simulink model "my_dom_model_statyczne"  (R2018a)
settings: Solver=VariableStepAuto  StartTime=0.0  StopTime=10.0  RelTol=1e-3
values from neighbouring files (symbols this model uses):
  c_p = 1000    [leveled_NL.m]    (also in leveled_state_space.m; leveled_transmitancja.m; my_dom.m; my_dom_state_space_script.m)
  C_vp = c_p*ro_p*V_p    (= 120000)    [leveled_NL.m]    (also in leveled_state_space.m; leveled_transmitancja.m; my_dom.m; my_dom_state_space_script.m)
  C_vw = c_p*ro_p*V_w    (= 1200000)    [leveled_NL.m]    (also in leveled_state_space.m; leveled_transmitancja.m; my_dom.m; my_dom_state_space_script.m)
  K_1 = K_matrix(1,1)    [leveled_NL.m]    (also in leveled_state_space.m; leveled_transmitancja.m; my_dom.m; my_dom_state_space_script.m)
  K_p = p*K_w    [leveled_NL.m]    (also in leveled_state_space.m; leveled_transmitancja.m; my_dom.m; my_dom_state_space_script.m)
  K_w = K_matrix(2,1)    [leveled_NL.m]    (also in leveled_state_space.m; leveled_transmitancja.m; my_dom.m; my_dom_state_space_script.m)
  ro_p = 1.2    [leveled_NL.m]    (also in leveled_state_space.m; leveled_transmitancja.m; my_dom.m; my_dom_state_space_script.m)
  slope_f_p = 0    [my_dom_statyczne.m]
  slope_T_z = 0    [my_dom_statyczne.m]
  slope_T_zew = 0.00001    (= 1e-05)    [my_dom_statyczne.m]
  T_pN = 19    [leveled_NL.m]    (also in leveled_state_space.m; leveled_transmitancja.m; my_dom.m; my_dom_state_space_script.m)
  T_wewN = 21    [leveled_NL.m]    (also in leveled_state_space.m; leveled_transmitancja.m; my_dom.m; my_dom_state_space_script.m)
libraries: simulink x3
settings Model: Creator=johnb  LastModifiedBy=johnb

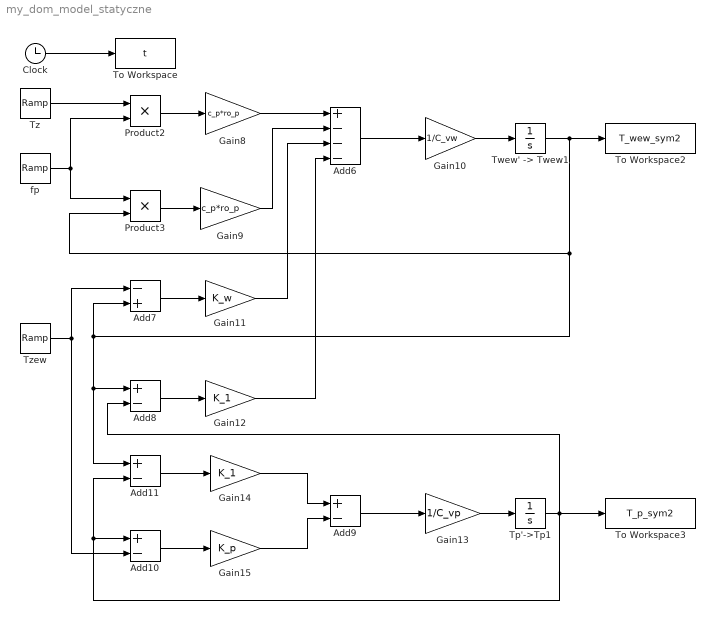
== system my_dom_model_statyczne ==
  Add{8..11} (4 alike) : Sum  Inputs=+-
  Add6 : Sum  Inputs=+---
  Add7 : Sum  Inputs=-+
  Clock : Clock
  Gain10 : Gain  Gain=1/C_vw
  Gain11 : Gain  Gain=K_w
  Gain12 : Gain  Gain=K_1
  Gain13 : Gain  Gain=1/C_vp
  Gain14 : Gain  Gain=K_1
  Gain15 : Gain  Gain=K_p
  Gain8 : Gain  Gain=c_p*ro_p
  Gain9 : Gain  Gain=c_p*ro_p
  Product2 : Product
  Product3 : Product
  To Workspace : ToWorkspace  VariableName=t  SampleTime=-1
  To Workspace2 : ToWorkspace  VariableName=T_wew_sym2  SampleTime=-1
  To Workspace3 : ToWorkspace  VariableName=T_p_sym2  SampleTime=-1
  Tp'->Tp1 : Integrator  InitialCondition=T_pN
  "Twew' -> Twew1" : Integrator  InitialCondition=T_wewN
  Tz : simulink/Sources/Ramp  slope=slope_T_z  start=0  InitialOutput=0
  Tzew : simulink/Sources/Ramp  slope=slope_T_zew  start=0  InitialOutput=0
  fp : simulink/Sources/Ramp  slope=slope_f_p  start=0  InitialOutput=0
  wires:
  Clock/1 -> To Workspace/1
  Gain12/1 -> Add6/4
  Add7/1 -> Gain11/1
  Gain13/1 -> Tp'->Tp1/1
  "Twew' -> Twew1"/1 -> To Workspace2/1, Add11/1, Add8/1, Add7/2, Product3/2
  Add8/1 -> Gain12/1
  fp/1 -> Product3/1, Product2/2
  Product2/1 -> Gain8/1
  Add10/1 -> Gain15/1
  Add9/1 -> Gain13/1
  Add11/1 -> Gain14/1
  Gain9/1 -> Add6/2
  Gain15/1 -> Add9/2
  Gain8/1 -> Add6/1
  Tzew/1 -> Add7/1, Add10/2
  Gain11/1 -> Add6/3
  Gain10/1 -> "Twew' -> Twew1"/1
  Product3/1 -> Gain9/1
  Add6/1 -> Gain10/1
  Tp'->Tp1/1 -> Add8/2, To Workspace3/1, Add11/2, Add10/1
  Gain14/1 -> Add9/1
  Tz/1 -> Product2/1
